simulink model "lab3_linear"  (R2023b)
settings: Solver=VariableStepAuto  StartTime=0.0  StopTime=10.0  RelTol=1e-3
values from neighbouring files (symbols this model uses):
  A = double(subs(J1, [x;u], [x_bar;u_bar]))    [lab3.m]
  B = double(subs(J2, [x;u], [x_bar;u_bar]))    [lab3.m]
  K = -K_lqr2    [lab3.m]
  x0 = 2*[0; 0; pi/24; 0]    [lab3.m]
settings Model: Creator=Darrian  LastModifiedBy=Darrian

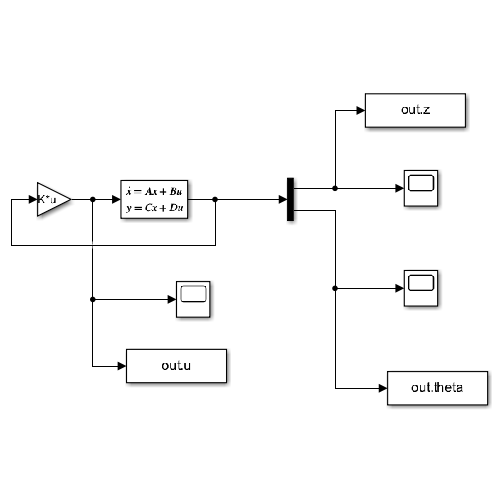
[thumbnail: Simulink's stored preview of the top-level diagram]
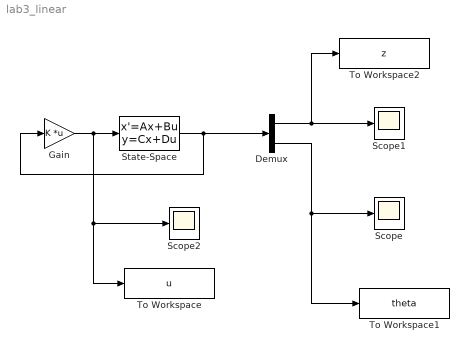
== system lab3_linear ==
  Demux : Demux  Outputs=2
  Gain : Gain  Gain=K  Multiplication=Matrix(K*u)
  Scope : Scope
  Scope1 : Scope
  Scope2 : Scope
  State-Space : StateSpace  A=A  B=B  C=eye(4)  D=zeros(4,1)  InitialCondition=x0
  To Workspace : ToWorkspace  VariableName=u  SaveFormat=Timeseries  SampleTime=-1
  To Workspace1 : ToWorkspace  VariableName=theta  SaveFormat=Timeseries  SampleTime=-1
  To Workspace2 : ToWorkspace  VariableName=z  SaveFormat=Timeseries  SampleTime=-1
  wires:
  Gain/1 -> To Workspace/1, Scope2/1, State-Space/1
  State-Space/1 -> Gain/1, Demux/1
  Demux/1 -> To Workspace2/1, Scope1/1
  Demux/2 -> To Workspace1/1, Scope/1
